simulink model "etc_with_bus"  (R2022b)
settings: Solver=ode45  StartTime=0.0  StopTime=10.0  RelTol=1e-3  EnableMultiTasking=on
PreLoadFcn:
  | load allParamValues
undefined symbols (not defined in the file): degConv, J, Kd, Km, Ks, theta_eq
settings Model: Creator=jrivitus  LastModifiedBy=bensweet
settings SolverCC: AlgebraicLoopSolver=TrustRegion
settings DataIOCC: LimitDataPoints=on  SaveFormat=Array  ReturnWorkspaceOutputs=off
settings OptimizationCC: ExpressionDepthLimit=2147483647  LifeSpan=inf
settings DebuggingCC: UnconnectedInputMsg=warning  UnconnectedOutputMsg=warning  UnconnectedLineMsg=warning  PregeneratedLibrarySubsystemCodeDiagnostic=none  SFMachineParentedDataDiag=warning
settings HardwareCC: ProdBitPerPointer=32  ProdBitPerSizeT=32  ProdBitPerPtrDiffT=32  ProdLargestAtomicFloat=None  ProdIntDivRoundTo=Undefined  ProdEndianess=Unspecified  ProdWordSize=32  ProdHWDeviceType=32-bit Generic
settings ModelReferenceCC: EnableRefExpFcnMdlSchedulingChecks=on  PropagateSignalLabelsOutOfModel=off
settings SFSimCC: SimUseLocalCustomCode=off
settings RTWCC: RTWUseLocalCustomCode=off  DLArmComputeVersion=19.05
settings CodeAppCC: StateflowObjectComments=on
settings GRTTargetCC: TargetLangStandard=C89/C90 (ANSI)  CombineOutputUpdateFcns=off  GRTInterface=on
settings ConfigComp: CovMetricSettings=dw  CovSaveCumulativeToWorkspaceVar=on  CovSaveSingleToWorkspaceVar=on  CovExternalEMLEnable=off  CovSFcnEnable=off

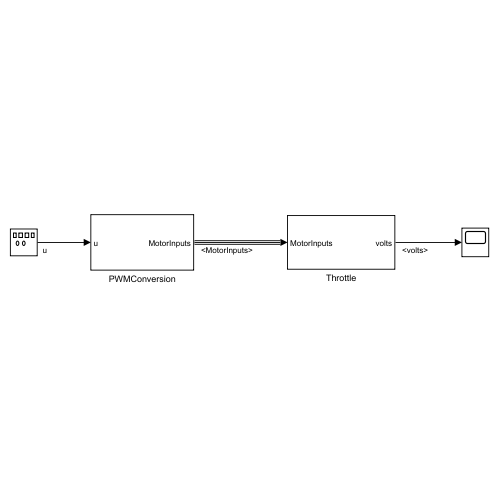
[thumbnail: Simulink's stored preview of the top-level diagram]
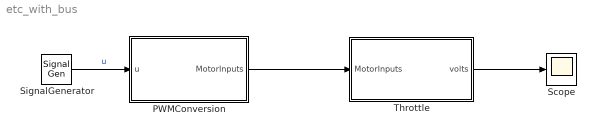
== system etc_with_bus ==
  PWMConversion : Subsystem
  Scope : Scope
  SignalGenerator : SignalGenerator  WaveForm=square  Amplitude=0.1
  Throttle : Subsystem
  wires:
  SignalGenerator/1 -> PWMConversion/1(u)  "u"
  PWMConversion/1(MotorInputs) -> Throttle/1(MotorInputs)
  Throttle/1(volts) -> Scope/1

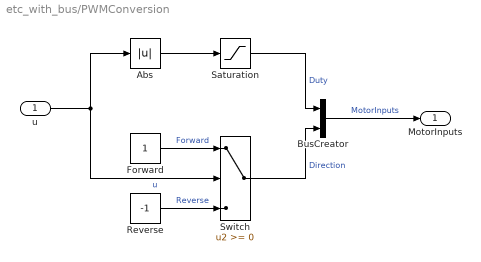
== system etc_with_bus/PWMConversion ==
  u : Inport
  Abs : Abs  SaturateOnIntegerOverflow=off
  BusCreator : BusCreator  Inputs=2
  Forward : Constant  OutDataTypeStr=double
  Reverse : Constant  Value=-1  OutDataTypeStr=double
  Saturation : Saturate  UpperLimit=1  LowerLimit=0
      settings: AttributesFormatString=%<LowerLimit> < duty < %<UpperLimit>
  Switch : Switch  SaturateOnIntegerOverflow=off  InputSameDT=off
      settings: AttributesFormatString=Criteria: %<Criteria>\nThreshold: %<Threshold>
  MotorInputs : Outport  VectorParamsAs1DForOutWhenUnconnected=off
  wires:
  Abs/1 -> Saturation/1
  Saturation/1 -> BusCreator/1  "Duty"
  Switch/1 -> BusCreator/2  "Direction"
  Reverse/1 -> Switch/3  "Reverse"
  Forward/1 -> Switch/1  "Forward"
  u/1 -> Switch/2, Abs/1  "u"
  BusCreator/1 -> MotorInputs/1  "MotorInputs"

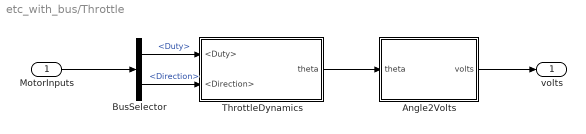
== system etc_with_bus/Throttle ==
  MotorInputs : Inport
  Angle2Volts : Subsystem
  BusSelector : BusSelector  OutputSignals=Duty,Direction
  ThrottleDynamics : Subsystem
  volts : Outport
  wires:
  MotorInputs/1 -> BusSelector/1
  Angle2Volts/1(volts) -> volts/1
  BusSelector/1 -> ThrottleDynamics/1(<Duty>)  "<Duty>"
  ThrottleDynamics/1(theta) -> Angle2Volts/1(theta)
  BusSelector/2 -> ThrottleDynamics/2(<Direction>)  "<Direction>"

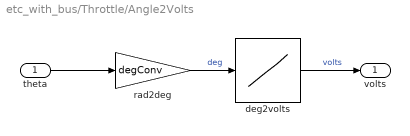
== system etc_with_bus/Throttle/Angle2Volts ==
  theta : Inport
  deg2volts : Lookup_n-D  NumberOfTableDimensions=1  BreakpointsForDimension1=[0 90]  Table=[0.5 4.5]  RndMeth=Simplest
  rad2deg : Gain  Gain=degConv  SaturateOnIntegerOverflow=on  OutDataTypeStr=Inherit: Same as input  ParamDataTypeStr=Inherit: Same as input
  volts : Outport  VectorParamsAs1DForOutWhenUnconnected=off
  wires:
  rad2deg/1 -> deg2volts/1  "deg"
  deg2volts/1 -> volts/1  "volts"
  theta/1 -> rad2deg/1

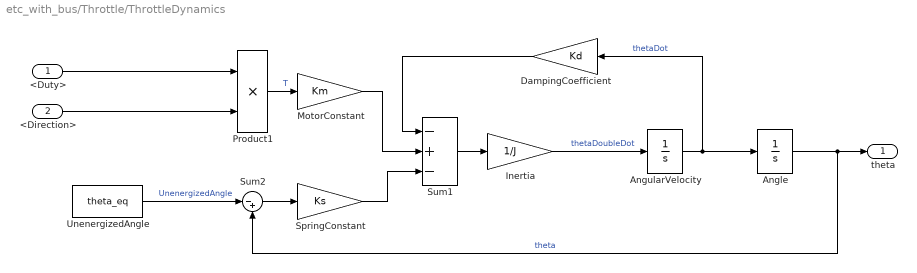
== system etc_with_bus/Throttle/ThrottleDynamics ==
  <Duty> : Inport
  <Direction> : Inport  Port=2
  Angle : Integrator  InitialCondition=pi/6  LimitOutput=on  UpperSaturationLimit=pi/2  LowerSaturationLimit=0
      settings: AttributesFormatString=Initial condition: %<InitialCondition>\n%<LowerSaturationLimit> <= theta <= %<UpperSaturationLimit>
  AngularVelocity : Integrator
      settings: AttributesFormatString=Initial condition: %<InitialCondition>
  DampingCoefficient : Gain  Gain=Kd  SaturateOnIntegerOverflow=on  OutDataTypeStr=Inherit: Same as input  ParamDataTypeStr=Inherit: Same as input
  Inertia : Gain  Gain=1/J  SaturateOnIntegerOverflow=on  OutDataTypeStr=Inherit: Same as input  ParamDataTypeStr=Inherit: Same as input
  MotorConstant : Gain  Gain=Km
  Product1 : Product  SaturateOnIntegerOverflow=on  OutDataTypeStr=Inherit: Same as first input
  SpringConstant : Gain  Gain=Ks  SaturateOnIntegerOverflow=on  OutDataTypeStr=Inherit: Same as input  ParamDataTypeStr=Inherit: Same as input
  Sum1 : Sum  Inputs=-+-  SaturateOnIntegerOverflow=on
  Sum2 : Sum  Inputs=|-+  SaturateOnIntegerOverflow=on
  UnenergizedAngle : Constant  Value=theta_eq
  theta : Outport
  wires:
  AngularVelocity/1 -> Angle/1, DampingCoefficient/1  "thetaDot"
  MotorConstant/1 -> Sum1/2
  Sum1/1 -> Inertia/1
  Product1/1 -> MotorConstant/1  "T"
  SpringConstant/1 -> Sum1/3
  DampingCoefficient/1 -> Sum1/1
  Inertia/1 -> AngularVelocity/1  "thetaDoubleDot"
  Sum2/1 -> SpringConstant/1
  UnenergizedAngle/1 -> Sum2/1  "UnenergizedAngle"
  Angle/1 -> theta/1, Sum2/2  "theta"
  <Duty>/1 -> Product1/1
  <Direction>/1 -> Product1/2
